simulink model "adaptive_backstepping_compliant_two_motor_k1_k2_k3_k4"  (R2022b)
settings: Solver=VariableStepAuto  StartTime=0.0  StopTime=2500  RelTol=1e-3
values from neighbouring files (symbols this model uses):
  Lamda = 1*eye(2)    [init.m]
settings Model: Creator=alexi  LastModifiedBy=alexi

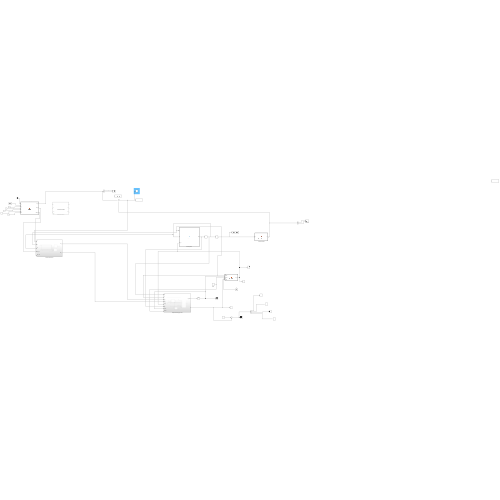
[thumbnail: Simulink's stored preview of the top-level diagram]
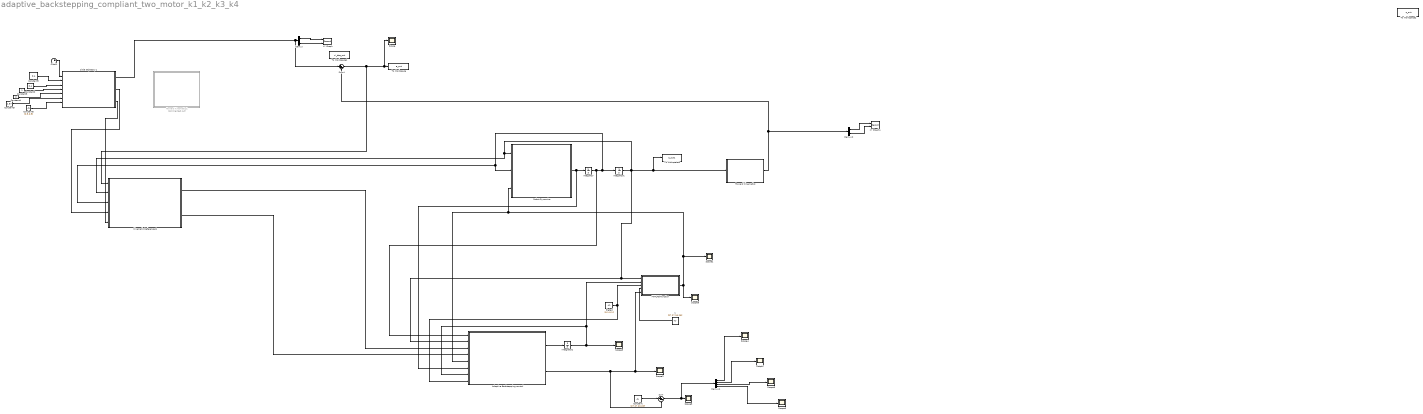
== system adaptive_backstepping_compliant_two_motor_k1_k2_k3_k4 ==
  Adaptive Backstepping control : Subsystem
  Clock1 : Clock
  Constant : Constant  Value=[27,27,20,20]'
  Constant2 : Constant  Value=0.4
  Constant3 : Constant
  Constant4 : Constant  Value=2
  Constant5 : Constant  Value=1.57
  Constant6 : Constant  Value=[0.5,0.5]
  Constant9 : Constant  Value=0.4
  Demux : Demux  Outputs=2
  Demux1 : Demux
  Demux2 : Demux  Outputs=2
  Forward Kinematics : MATLAB Function  TreatAsAtomicUnit=on
  Forward Kinematics1 : MATLAB Function  Commented=on  TreatAsAtomicUnit=on
  Integrator : Integrator  InitialCondition=[0,0]'
  Integrator1 : Integrator  InitialCondition=[0.1,0.1]'
  Integrator2 : Integrator  InitialCondition=[0.1,0.1]'
  Kinematic References1 : Subsystem
  MATLAB Function : MATLAB Function  TreatAsAtomicUnit=on
  Robot Dynamics : MATLAB Function  TreatAsAtomicUnit=on
  Scope{,1..9} (10 alike) : Scope
  Sum : Sum  Inputs=|+-
  Sum4 : Sum  Inputs=|+-
  To Workspace : ToWorkspace  VariableName=e_out  SaveFormat=Timeseries  SampleTime=-1
  To Workspace1 : ToWorkspace  VariableName=xi_des_out  SaveFormat=Timeseries  SampleTime=-1
  To Workspace2 : ToWorkspace  VariableName=q_out  SaveFormat=Timeseries  SampleTime=-1
  To Workspace3 : ToWorkspace  VariableName=q_out1  SaveFormat=Timeseries  SampleTime=-1
  XY Graph : Record  FileSettingsInternal="{\"entries\":[{\"content\":{\"excelSettings\":{\"content\":{},\"type\":\"Streamout.ExcelSettings\"}},\"type\":\"Streamout.FileSettingStorage\",\"uuid\":\"24894c47-d9c7-498f-abfd-cee5b240e213\"}],\"packageUris\":[\"http://schema.mathworks.com/mf0/streamout_blocks/R2020a\"],\"version\":\"1.0\"}"  Layout=[1 1]  SignalsInternal="{\"entries\":[{\"content\":{\"signals\":[{\"content\":{\"blockPath\":[\"adaptive_backstepping_compliant_two_motor_k1_k2_k3_k4/XY Graph\"],\"channel\":[],\"dimensions\":[1],\"domain\":\"adaptive_backstepping_compliant_two_motor_k1_k2_k3_k4/XY Graph\",\"lineColor\":\"#a2142f\",\"plots\":[1],\"port\":1,\"sid\":[\"\"],\"signalID\":46454,\"signalName\":\"Demux:1\"},\"type\":\"RecordBlkView.Signal\",\"uuid\":\"cc412ee4-e94f-46a1-a718-55c57284bfbf\"},{\"content\":{\"blockPath\":[\"adaptive_backstepping_compliant_two_motor_k1_k2_k3_k4/XY Graph\"],\"channel\":[],\"dimensions\":[1],\"domain\":\"adaptive_backstepping_compliant_two_motor_k1_k2_k3_k4/XY Graph\",\"lineColor\":\"#139fff\",\"plots\":[1],\"port\":2,\"sid\":[\"\"],\"signalID\":46458,\"signalName\":\"Demux:2\"},\"type\":\"RecordBlkView.Signal\",\"uuid\":\"b8ad076f-4be7-4864-9012-602b2fbfc63a\"}]},\"type\":\"RecordBlkView.InputSignals\",\"uuid\":\"adaf56c1-2b65-45f0-ab71-c739c7506d1d\"}],\"packageUris\":[\"http://schema.mathworks.com/mf0/streamout_blocks/R2020a\"],\"version\":\"1.0\"}"  VisualizationBindings="{\"xyplotplugin\":{\"info\":[{\"series\":[{\"bindingParametersList\":[{\"parameter\":\"X-Axis\",\"signalID\":46454,\"signalName\":\"Demux:1\"},{\"parameter\":\"Y-Axis\",\"signalID\":46458,\"signalName\":\"Demux:2\"}],\"seriesID\":51887}],\"subplotID\":1}]}}"  CompatibilityTag=XY
  XY Graph1 : Record  FileSettingsInternal="{\"entries\":[{\"content\":{\"excelSettings\":{\"content\":{},\"type\":\"Streamout.ExcelSettings\"}},\"type\":\"Streamout.FileSettingStorage\",\"uuid\":\"f96bc0ea-1990-46e8-8ada-27f034c0f8be\"}],\"packageUris\":[\"http://schema.mathworks.com/mf0/streamout_blocks/R2020a\"],\"version\":\"1.0\"}"  Layout=[1 1]  SignalsInternal="{\"entries\":[{\"content\":{\"signals\":[{\"content\":{\"blockPath\":[\"adaptive_backstepping_compliant_two_motor_k1_k2_k3_k4/XY Graph1\"],\"channel\":[],\"dimensions\":[1],\"domain\":\"adaptive_backstepping_compliant_two_motor_k1_k2_k3_k4/XY Graph1\",\"lineColor\":\"#a2142f\",\"plots\":[1],\"port\":1,\"sid\":[\"\"],\"signalID\":46462,\"signalName\":\"Demux2:1\"},\"type\":\"RecordBlkView.Signal\",\"uuid\":\"3c8b16c2-7a27-4da6-a3e6-925b9a20117b\"},{\"content\":{\"blockPath\":[\"adaptive_backstepping_compliant_two_motor_k1_k2_k3_k4/XY Graph1\"],\"channel\":[],\"dimensions\":[1],\"domain\":\"adaptive_backstepping_compliant_two_motor_k1_k2_k3_k4/XY Graph1\",\"lineColor\":\"#139fff\",\"plots\":[1],\"port\":2,\"sid\":[\"\"],\"signalID\":46466,\"signalName\":\"Demux2:2\"},\"type\":\"RecordBlkView.Signal\",\"uuid\":\"c1f8ee4f-bdc0-4cee-940d-221abbc463be\"}]},\"type\":\"RecordBlkView.InputSignals\",\"uuid\":\"88e04999-40eb-4bc6-8df6-5d9971d0041c\"}],\"packageUris\":[\"http://schema.mathworks.com/mf0/streamout_blocks/R2020a\"],\"version\":\"1.0\"}"  VisualizationBindings="{\"xyplotplugin\":{\"info\":[{\"series\":[{\"bindingParametersList\":[{\"parameter\":\"X-Axis\",\"signalID\":46462,\"signalName\":\"Demux2:1\"},{\"parameter\":\"Y-Axis\",\"signalID\":46466,\"signalName\":\"Demux2:2\"}],\"seriesID\":8208}],\"subplotID\":1}]}}"  CompatibilityTag=XY
  circle trajectory1 : MATLAB Function  TreatAsAtomicUnit=on
  k : Constant  Value=[27,27,20,20]'
  thetad : Constant  Value=[0.1,0.1]'
  wires:
  MATLAB Function/1(tau_el) -> Scope1/1, Robot Dynamics/3(tau_el), Adaptive Backstepping control/5(tau_el), Scope9/1
  thetad/1 -> Adaptive Backstepping control/8(thetad), MATLAB Function/3(thetad)
  Robot Dynamics/1(ddq) -> Adaptive Backstepping control/6(ddq), Integrator/1
  Demux/1 -> XY Graph/1
  Kinematic References1/2(ddq_r) -> Adaptive Backstepping control/4(ddq_r)
  Adaptive Backstepping control/1(d_thetas) -> Integrator2/1
  Kinematic References1/1(dq_r) -> Adaptive Backstepping control/3(dq_r)
  Integrator/1 -> Adaptive Backstepping control/1(dq), Integrator1/1, Robot Dynamics/2(dq), Kinematic References1/3(dq)  "dq"
  Forward Kinematics/1(xi) -> Demux2/1, Sum4/2  "xi"
  Integrator2/1 -> Adaptive Backstepping control/7(thetas), MATLAB Function/2(thetas), Scope5/1
  Sum4/1 -> Scope/1, To Workspace/1, Kinematic References1/1(e)
  Integrator1/1 -> Adaptive Backstepping control/2(q), MATLAB Function/1(q), Forward Kinematics/1(q), To Workspace3/1, Kinematic References1/2(q), Robot Dynamics/1(q)  "q"
  Adaptive Backstepping control/2(pi) -> MATLAB Function/5(pi_hat), Scope2/1, Sum/2
  Constant/1 -> Sum/1
  Sum/1 -> Demux1/1, Scope3/1
  Constant3/1 -> circle trajectory1/4(a)
  Constant4/1 -> circle trajectory1/5(b)
  Constant9/1 -> circle trajectory1/2(A)
  Constant2/1 -> circle trajectory1/3(B)
  Clock1/1 -> circle trajectory1/1(t)
  Constant6/1 -> circle trajectory1/7(p0)
  Constant5/1 -> circle trajectory1/6(d)
  Demux/2 -> XY Graph/2
  k/1 -> MATLAB Function/4(pi)
  Demux1/1 -> Scope4/1
  Demux1/2 -> Scope7/1
  Demux2/1 -> XY Graph1/1
  Demux2/2 -> XY Graph1/2
  Demux1/4 -> Scope6/1
  Demux1/3 -> Scope8/1
  circle trajectory1/1(xi_des) -> Sum4/1, Demux/1
  circle trajectory1/2(dxi_des) -> Kinematic References1/4(dxi_des)
  circle trajectory1/3(ddxi_des) -> Kinematic References1/5(ddxi_des)

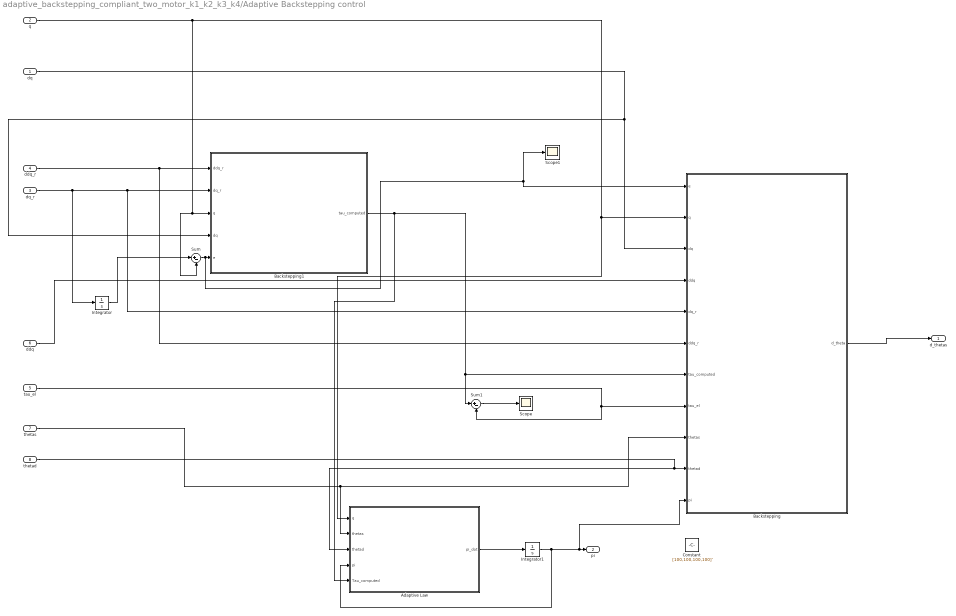
== system adaptive_backstepping_compliant_two_motor_k1_k2_k3_k4/Adaptive Backstepping control ==
  dq : Inport
  q : Inport  Port=2
  dq_r : Inport  Port=3
  ddq_r : Inport  Port=4
  tau_el : Inport  Port=5
  ddq : Inport  Port=6
  thetas : Inport  Port=7
  thetad : Inport  Port=8
  Adaptive Law : MATLAB Function  TreatAsAtomicUnit=on
  Backstepping : MATLAB Function  TreatAsAtomicUnit=on
  Backstepping1 : MATLAB Function  TreatAsAtomicUnit=on
  Constant : Constant  Value=[100,100,100,100]'
  Integrator : Integrator  InitialCondition=[0.1,0.1]'
  Integrator1 : Integrator  InitialCondition=[35,35,30,30]'
  Scope : Scope
  Scope1 : Scope
  Sum : Sum  Inputs=|+-
  Sum1 : Sum  Inputs=|+-
  d_thetas : Outport
  pi : Outport  Port=2
  wires:
  dq_r/1 -> Integrator/1, Backstepping1/2(dq_r), Backstepping/5(dq_r)
  q/1 -> Adaptive Law/1(q), Backstepping/2(q), Backstepping1/3(q), Sum/2
  Backstepping1/1(tau_computed) -> Adaptive Law/5(Tau_computed), Sum1/1, Backstepping/7(tau_computed)
  tau_el/1 -> Backstepping/8(tau_el), Sum1/2
  ddq_r/1 -> Backstepping/6(ddq_r), Backstepping1/1(ddq_r)
  dq/1 -> Backstepping1/4(dq), Backstepping/3(dq)
  Backstepping/1(d_theta) -> d_thetas/1
  ddq/1 -> Backstepping/4(ddq)
  thetas/1 -> Backstepping/9(thetas), Adaptive Law/2(thetas)
  Integrator/1 -> Sum/1
  Sum/1 -> Scope1/1, Backstepping/1(e), Backstepping1/5(e)
  thetad/1 -> Adaptive Law/3(thetad), Backstepping/10(thetad)
  Sum1/1 -> Scope/1
  Integrator1/1 -> Backstepping/11(pi), pi/1, Adaptive Law/4(pi)
  Adaptive Law/1(pi_dot) -> Integrator1/1

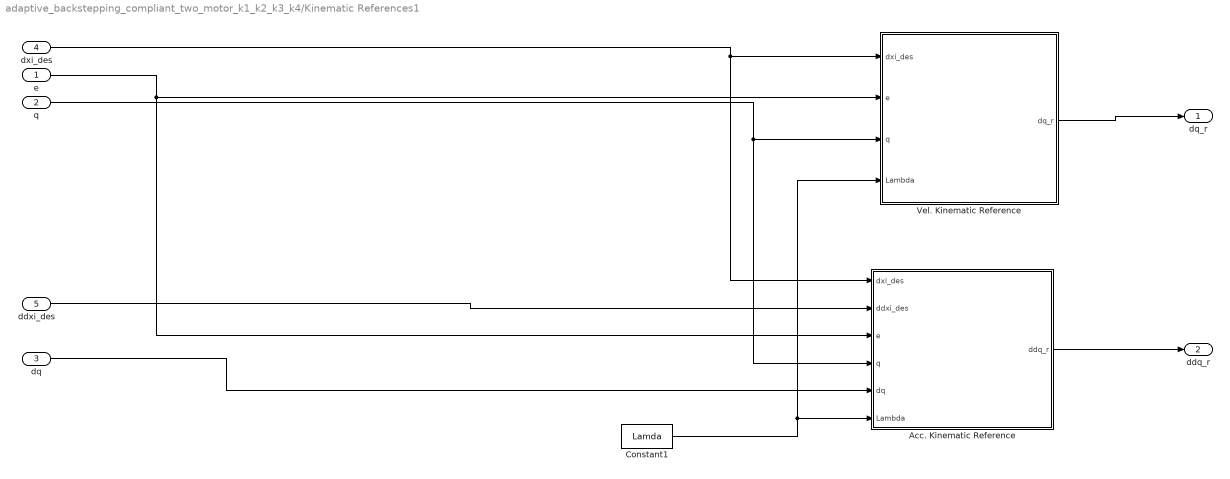
== system adaptive_backstepping_compliant_two_motor_k1_k2_k3_k4/Kinematic References1 ==
  e : Inport
  q : Inport  Port=2
  dq : Inport  Port=3
  dxi_des : Inport  Port=4
  ddxi_des : Inport  Port=5
  Acc. Kinematic Reference : MATLAB Function  TreatAsAtomicUnit=on
  Constant1 : Constant  Value=Lamda
  "Vel. Kinematic Reference " : MATLAB Function  TreatAsAtomicUnit=on
  dq_r : Outport  VectorParamsAs1DForOutWhenUnconnected=off
  ddq_r : Outport  Port=2  VectorParamsAs1DForOutWhenUnconnected=off
  wires:
  ddxi_des/1 -> Acc. Kinematic Reference/2(ddxi_des)
  e/1 -> Acc. Kinematic Reference/3(e), "Vel. Kinematic Reference "/2(e)
  dxi_des/1 -> Acc. Kinematic Reference/1(dxi_des), "Vel. Kinematic Reference "/1(dxi_des)
  Constant1/1 -> "Vel. Kinematic Reference "/4(Lambda), Acc. Kinematic Reference/6(Lambda)
  "Vel. Kinematic Reference "/1(dq_r) -> dq_r/1
  dq/1 -> Acc. Kinematic Reference/5(dq)
  q/1 -> Acc. Kinematic Reference/4(q), "Vel. Kinematic Reference "/3(q)
  Acc. Kinematic Reference/1(ddq_r) -> ddq_r/1

== matlab function adaptive_backstepping_compliant_two_motor_k1_k2_k3_k4/Forward Kinematics ==
  data: q input; xi output
function xi  = RR_forward_kinematics(q)

    q1 = q(1);
    q2 = q(2);

    a1 = 1;
    a2 = 1;

    p0 = [0;0];
    p1 = [a1*cos(q1); a1*sin(q1)];
    xi = p1+[a2*cos(q1+q2);a2*sin(q1+q2)];
end

== matlab function adaptive_backstepping_compliant_two_motor_k1_k2_k3_k4/Adaptive Backstepping control/Adaptive Law ==
  data: q input; thetas input; thetad input; pi input; pi_dot output; Tau_computed input; R parameter
function pi_dot = fcn(q,thetas,thetad,pi,Tau_computed,R)
Kc = 100*eye(2);
Y = RR_Regression_Matrix_two_motors_k1_k2_k3_k4(q,thetas,thetad);
pi_dot = inv(R)*(Y'*Kc*Tau_computed-Y'*Kc*Y*pi);

== matlab function adaptive_backstepping_compliant_two_motor_k1_k2_k3_k4/Kinematic References1/Acc. Kinematic Reference ==
  data: dxi_des input; ddq_r output; ddxi_des input; e input; q input; dq input; Lambda input
function ddq_r = acc_kinematic_reference(dxi_des, ddxi_des, e, q, dq, Lambda)

coder.extrinsic('disp');

J = zeros(2,2);
dJ = zeros(2,2);

dq1 = dq(1);
dq2 = dq(2);

q1 = q(1);
q2 = q(2);

a1 = 1;
a2 = 1;

% Computing jacobian and derivative
J = [-a2*sin(q1 + q2) - a1*sin(q1), -a2*sin(q1 + q2);
      a2*cos(q1 + q2) + a1*cos(q1),  a2*cos(q1 + q2)];

dJ = [-a2*cos(q1 + q2)*(dq1 + dq2)-a1*cos(q1)*dq1, -a2*cos(q1 + q2)*(dq1 + dq2);
    -a2*sin(q1 + q2)*(dq1 + dq2)-a1*sin(q1)*dq1, -a2*sin(q1 + q2)*(dq1 + dq2)];

ddq_r = inv(J) * (ddxi_des + Lambda*dxi_des - Lambda*J*dq) ...
- inv(J)*dJ*inv(J)*(dxi_des + Lambda*e);
end

== matlab function adaptive_backstepping_compliant_two_motor_k1_k2_k3_k4/Kinematic References1/Vel. Kinematic Reference  ==
  data: dxi_des input; dq_r output; e input; q input; Lambda input
function dq_r = vel_kinematic_reference(dxi_des, e, q, Lambda)
a1 = 1;
a2 = 1;

q1 = q(1);
q2 = q(2);

% Computing jacobian
J = [-a2*sin(q1 + q2) - a1*sin(q1), -a2*sin(q1 + q2);
      a2*cos(q1 + q2) + a1*cos(q1),  a2*cos(q1 + q2)];

dq_r = inv(J) * (dxi_des + Lambda*e);
end

== matlab function adaptive_backstepping_compliant_two_motor_k1_k2_k3_k4/Forward Kinematics1 ==
  data: q input; xi output; dq input; ddq input; dxi output; ddxi output
function [xi,dxi,ddxi]   = RR_forward_kinematics(q,dq,ddq)

    q1 = q(1);
    q2 = q(2);

    a1 = 1;
    a2 = 1;

    p0 = [0;0];
    p1 = [a1*cos(q1); a1*sin(q1)];
    xi = p1+[a2*cos(q1+q2);a2*sin(q1+q2)];
    dxi = [-a1*sin(q1)*dq(1);a1*cos(q1)*dq(1)]+[-a2*sin(q1+q2)*(dq(1)+dq(2)); a2*cos(q1+q2)*(dq(1)+dq(2))];
    ddxi = [-a1*cos(q1)*dq(1)^2-a1*sin(q1)*ddq(1);-a1*sin(q1)*dq(1)^2+a1*cos(q1)*ddq(1)]+[-a2*cos(q1+q2)*(dq(1)+dq(2))^2-a2*sin(q1+q2)*(ddq(1)+ddq(2)); -a2*sin(q1+q2)*(dq(1)+dq(2))^2 + a2*cos(q1+q2)*(ddq(1)+ddq(2))];
end

== matlab function adaptive_backstepping_compliant_two_motor_k1_k2_k3_k4/Adaptive Backstepping control/Backstepping1 ==
  data: ddq_r input; dq_r input; q input; dq input; e input; tau_computed output
function tau_computed  = computed_torque(ddq_r,dq_r,q,dq,e)

coder.extrinsic('disp');
rel_err = 0;

de = dq_r-dq;
Kp = 35;
Kv = 12;

% Get dynamic matrices
B = RR_mass_matrix(q);
C = RR_coriolis_matrix(q,dq);
G = RR_gravity_vector(q);

% Adding uncertainty
B = B.*(1 + rel_err);
C = C.*(1 + rel_err);
G = G.*(1 + rel_err);

% Control law
tau_computed = -(B*ddq_r+C*dq+G+B*Kp*e+B*Kv*de);

== matlab function adaptive_backstepping_compliant_two_motor_k1_k2_k3_k4/circle trajectory1 ==
  data: t input; xi_des output; A input; B input; a input; b input; d input; p0 input; dxi_des output; ddxi_des output
function [xi_des,dxi_des,ddxi_des]  = lissajous(t,A,B,a,b,d,p0)

xi_des = [A*sin(a*t+d); B*sin(b*t)] + p0;
dxi_des = [A*a*cos(a*t+d); B*b*cos(b*t)];
ddxi_des = [-A*a^2*sin(a*t+d); -B*b^2*sin(b*t)];

% R = 0.2;
% xi_des = [R*( - sin(2*t+pi)); R*(1-cos(2*t+pi))+p0];
% dxi_des = [- 2*R*cos(2*t+pi); 2*R*sin(2*t+pi)];
% ddxi_des = [4*R*sin(2*t+pi); 4*R*cos(2*t+pi)];

% omega = 0.001;
% x0 = 0;
% y0 = 0;
% A = 1;
% B = 3;
% q1 = A*cos(omega*t);
% dq1 = -A*omega*sin(omega*t);
% ddq1 =  -A*omega^2*cos(omega*t);
% q2 = B*cos(2*omega*t) + y0;
% dq2 = -B*2*omega*sin(2*omega*t);
% ddq2 = -B*2*omega^2*cos(omega*t);
% q = [q1;q2];
% dq = [dq1;dq2];
% ddq = [ddq1;ddq2];

== matlab function adaptive_backstepping_compliant_two_motor_k1_k2_k3_k4/MATLAB Function ==
  data: q input; tau_el output; thetas input; thetad input; pi input; pi_hat input
function tau_el  = tau_elastica(q,thetas,thetad,pi,pi_hat)
% k = 0.1;
% a = 9;
k1 = pi(1);
k2 = pi(2);
k3 = pi(3);
k4 = pi(4);

% k1_hat = pi_hat(1);
% k2_hat = pi_hat(2);
% k3_hat = pi_hat(3);
% k4_hat = pi_hat(4);

tau_el1 = k1*(q(1)-thetas(1)-thetad(1)) + k2*(q(1) - thetas(1) + thetad(1)) + k1*(q(1)-thetas(1) - thetad(1))^2 + k2*(q(1)-thetas(1) + thetad(1))^2 + k1*(q(1)-thetas(1) - thetad(1))^3 + k2*(q(1)-thetas(1) + thetad(1))^3 + k1*(q(1)-thetas(1) - thetad(1))^4 + k2*(q(1)-thetas(1) + thetad(1))^4;
tau_el2 = k3*(q(2)-thetas(2)-thetad(2)) + k4*(q(2) - thetas(2) + thetad(2)) + k3*(q(2)-thetas(2) - thetad(2))^2 + k4*(q(2)-thetas(2) + thetad(2))^2 + k3*(q(2)-thetas(2) - thetad(2))^3 + k4*(q(2)-thetas(2) + thetad(2))^3 + k3*(q(2)-thetas(2) - thetad(2))^4 + k4*(q(2)-thetas(2) + thetad(2))^4;
tau_el = [tau_el1;tau_el2];
% 
% tau_el1_hat = k1_hat*(q(1)-thetas(1)-thetad(1)) + k1_hat*(q(1) - thetas(1) + thetad(1)) + k2_hat*(q(1)-thetas(1) - thetad(1))^2 + k2_hat*(q(1)-thetas(1) + thetad(1))^2 + k3_hat*(q(1)-thetas(1) - thetad(1))^3 + k3_hat*(q(1)-thetas(1) + thetad(1))^3 + k4_hat*(q(1)-thetas(1) - thetad(1))^4 + k4_hat*(q(1)-thetas(1) + thetad(1))^4;
% tau_el2_hat = k1_hat*(q(2)-thetas(2)-thetad(2)) + k1_hat*(q(2) - thetas(2) + thetad(2)) + k2_hat*(q(2)-thetas(2) - thetad(2))^2 + k2_hat*(q(2)-thetas(2) + thetad(2))^2 + k3_hat*(q(2)-thetas(2) - thetad(2))^3 + k3_hat*(q(2)-thetas(2) + thetad(2))^3 + k4_hat*(q(2)-thetas(2) - thetad(2))^4 + k4_hat*(q(2)-thetas(2) + thetad(2))^4;
% tau_el_hat = [tau_el1_hat;tau_el2_hat];

== matlab function adaptive_backstepping_compliant_two_motor_k1_k2_k3_k4/Adaptive Backstepping control/Backstepping ==
  data: e input; q input; dq input; ddq input; dq_r input; ddq_r input; tau_computed input; tau_el input; d_theta output; thetas input; thetad input; pi input
function d_theta  = backstepping(e,q,dq,ddq,dq_r,ddq_r,tau_computed,tau_el,thetas,thetad,pi)

coder.extrinsic('disp');
rel_err = 0;
de = dq_r-dq;
dde = ddq_r-ddq;
P = 0.9*eye(2);
K = 0.1;
Kc = 100;
Kp = 35;
Kv = 12;
a = 9;

k1_hat = pi(1);
k2_hat = pi(2);
k3_hat = pi(3);
k4_hat = pi(4);

% k1_hat = 200;
% k1_hat = 200;
% k2_hat = 200;
% k2_hat = 200;

% Get dynamic matrices
B = RR_mass_matrix(q);
C = RR_coriolis_matrix(q,dq);
G = RR_gravity_vector(q);

% Adding uncertainty
B = B.*(1 + rel_err);
C = C.*(1 + rel_err);
G = G.*(1 + rel_err);
g = [zeros(2,2); pinv(B)];
d_tau = C*dde-B*Kv*dde-B*Kp*de;

a1 = 1;
a2 = 1;

% Control law
%d_theta = B*ddq_r + C*dq_r + G + Ks*de + J.'*e;
Vx1 = [e'*Kp,de'];

l1 = -k1_hat - k2_hat - 2*k1_hat*(q(1)-thetas(1)-thetad(1)) - 2*k2_hat*(q(1)-thetas(1) + thetad(1)) - 3*k1_hat*(q(1)-thetas(1)-thetad(1))^2 - 3*k2_hat*(q(1)-thetas(1)+thetad(1))^2 - 4*k1_hat*(q(1)-thetas(1)-thetad(1))^3 - 4*k2_hat*(q(1)-thetas(1)+thetad(1))^3;
l2 = -k3_hat - k4_hat - 2*k3_hat*(q(2)-thetas(2)-thetad(2)) - 2*k4_hat*(q(2)-thetas(2) + thetad(2)) - 3*k3_hat*(q(2)-thetas(2)-thetad(2))^2 - 3*k4_hat*(q(2)-thetas(2)+thetad(2))^2 - 4*k3_hat*(q(2)-thetas(2)-thetad(2))^3 - 4*k4_hat*(q(2)-thetas(2)+thetad(2))^3;


l = [l1 0; 0 l2];


h1 = k1_hat*dq(1) + k2_hat*dq(1) + 2*k1_hat*(q(1)-thetas(1)-thetad(1))*dq(1) + 2*k2_hat*(q(1)-thetas(1)+thetad(1))*dq(1) + 3*k1_hat*dq(1)*(q(1)-thetas(1)-thetad(1))^2 + 3*k2_hat*dq(1)*(q(1)-thetas(1)+thetad(1))^2 + 4*k1_hat*dq(1)*(q(1)-thetas(1)-thetad(1))^3 + 4*k2_hat*dq(1)*(q(1)-thetas(1)+thetad(1))^3;
h2 = k3_hat*dq(2) + k4_hat*dq(2) + 2*k3_hat*(q(2)-thetas(2)-thetad(2))*dq(2) + 2*k4_hat*(q(2)-thetas(2)+thetad(2))*dq(2) + 3*k3_hat*dq(2)*(q(2)-thetas(2)-thetad(2))^2 + 3*k4_hat*dq(2)*(q(2)-thetas(2)+thetad(2))^2 + 4*k3_hat*dq(2)*(q(2)-thetas(2)-thetad(2))^3 + 4*k4_hat*dq(2)*(q(2)-thetas(2)+thetad(2))^3;

h = [h1;h2];

v = d_tau+pinv(P)*(Kc*(tau_computed-tau_el)-g'*Vx1');
d_theta = inv(l)*(v-h);

== matlab function adaptive_backstepping_compliant_two_motor_k1_k2_k3_k4/Robot Dynamics ==
  data: q input; dq input; tau_el input; ddq output
function ddq = inverse_dynamics(q,dq, tau_el)

% Get dynamic matrices
B = RR_mass_matrix(q);
C = RR_coriolis_matrix(q,dq);
G = RR_gravity_vector(q);
ddq = pinv(B)*(-tau_el - C*dq - G);
